simulink model "simulation_3"  (R2023b)
settings: Solver=VariableStepAuto  StartTime=0.0  StopTime=10.0  RelTol=1e-3
model workspace (MAT data in the model file):
  L = Simulink.Parameter
  L.Value = 50
  L.DataType = 'auto'
  L.DocUnits = 'm'
  L.Complexity = 'real'
  L.Dimensions = [1 1]
  c = Simulink.Parameter
  c.Value = 340
  c.DataType = 'auto'
  c.DocUnits = 'm/s'
  c.Complexity = 'real'
  c.Dimensions = [1 1]
  n = Simulink.Parameter
  n.Value = Simulink.data.Expression
  n.Value.ExpressionString = "[2*pi*f*(L/c)]"
  n.DataType = 'auto'
  n.Complexity = 'real'
  n.Dimensions = -1
  v = 92.3997839291
settings Model: Creator=nurbi  LastModifiedBy=nurbi

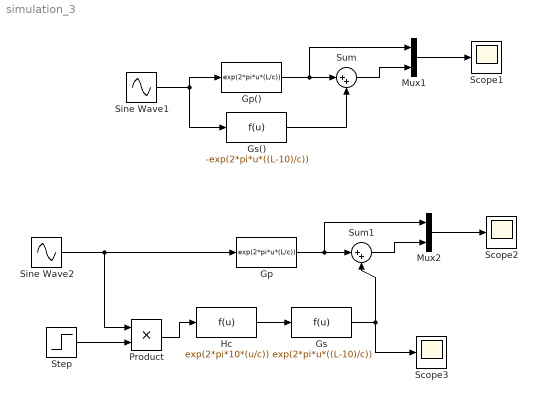
== system simulation_3 ==
  Gp : Fcn  Expr=exp(2*pi*u*(L/c))
  Gp() : Fcn  Expr=exp(2*pi*u*(L/c))
  Gs : Fcn  Expr=exp(2*pi*u*((L-10)/c))
  Gs() : Fcn  Expr=-exp(2*pi*u*((L-10)/c))
  Hc : Fcn  Expr=exp(2*pi*10*(u/c))
  Mux1 : Mux  Inputs=2
  Mux2 : Mux  Inputs=2
  Product : Product
  Scope1 : Scope
  Scope2 : Scope
  Scope3 : Scope
  Sine Wave1 : Sin  SampleTime=0
  Sine Wave2 : Sin  SampleTime=0
  Step : Step  SampleTime=0
  Sum : Sum  Inputs=|++
  Sum1 : Sum  Inputs=|++
  wires:
  Mux1/1 -> Scope1/1
  Sine Wave1/1 -> Gs()/1, Gp()/1
  Gp()/1 -> Mux1/1, Sum/1
  Gs()/1 -> Sum/2
  Sum/1 -> Mux1/2
  Mux2/1 -> Scope2/1
  Gp/1 -> Mux2/1, Sum1/1
  Sum1/1 -> Mux2/2
  Sine Wave2/1 -> Gp/1, Product/1
  Gs/1 -> Scope3/1, Sum1/2
  Hc/1 -> Gs/1
  Product/1 -> Hc/1
  Step/1 -> Product/2
